simulink model "PEMFC"  (Simulink 8.3)
settings: Solver=ode45  StartTime=5.0  StopTime=20.0  RelTol=1e-3
settings Model: Creator=Cindy  LastModifiedBy=Cindy
settings DataIOCC: SaveState=on  SignalLoggingName=sigsOut
settings DebuggingCC: SaveWithParameterizedLinksMsg=none  SignalResolutionControl=TryResolveAllWithWarning  SolverPrmCheckMsg=none  MultiTaskDSMMsg=warning  MultiTaskCondExecSysMsg=none  StateNameClashWarn=none
settings HardwareCC: TargetUnknown=on
settings RTWCC: IncludeERTFirstTime=on

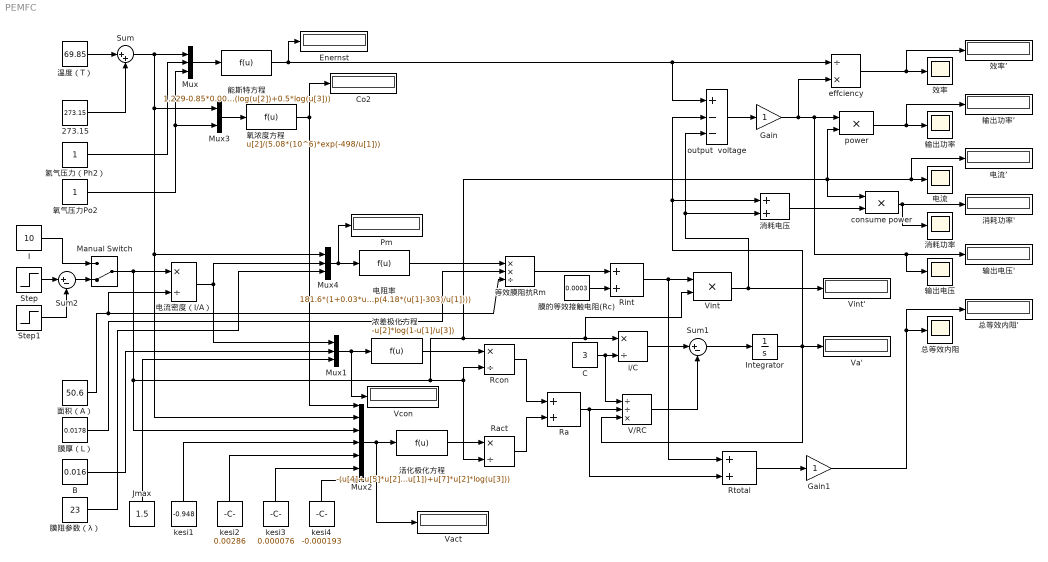
== system PEMFC ==
  273.15 : Constant  Value=273.15
  B : Constant  Value=0.016
  C : Constant  Value=3
  Co2 : Display
      settings: Format=short_e  Decimation=5
  Enernst : Display
      settings: Decimation=5
  Gain : Gain  SaturateOnIntegerOverflow=on  OutDataTypeStr=Inherit: Same as input  ParamDataTypeStr=Inherit: Same as input
  Gain1 : Gain  SaturateOnIntegerOverflow=on  OutDataTypeStr=Inherit: Same as input  ParamDataTypeStr=Inherit: Same as input
  I : Constant  Value=10
  Integrator : Integrator
  Jmax : Constant  Value=1.5
  Manual Switch : ManualSwitch  CurrentSetting=0
  Mux : Mux  Inputs=3
  Mux1 : Mux  Inputs=3
  Mux2 : Mux  Inputs=7
  Mux3 : Mux  Inputs=2
  Mux4 : Mux  Inputs=3
  Pm : Display
      settings: Decimation=5
  Ra : Sum  OutDataTypeStr=double
  Ract : Product  Inputs=*/  OutDataTypeStr=double
  Rcon : Product  Inputs=*/  OutDataTypeStr=double
  Rint : Sum  OutDataTypeStr=double
  Rtotal : Sum  OutDataTypeStr=double
  Step : Step  Time=10  Before=10  After=20  SampleTime=0
  Step1 : Step  Time=15  After=10  SampleTime=0
  Sum : Sum  Inputs=|++  SaturateOnIntegerOverflow=on
  Sum1 : Sum  Inputs=|+-  SaturateOnIntegerOverflow=on
  Sum2 : Sum  Inputs=|+-  SaturateOnIntegerOverflow=on
  V/RC : Product  Inputs=//*  OutDataTypeStr=double
  Va' : Display
      settings: Decimation=5
  Vact : Display
      settings: Decimation=5
  Vcon : Display
      settings: Decimation=5
  Vint : Product  SaturateOnIntegerOverflow=on  OutDataTypeStr=Inherit: Same as first input
  Vint' : Display
      settings: Decimation=5
  consume power : Product  SaturateOnIntegerOverflow=on  OutDataTypeStr=Inherit: Same as first input
  effciency : Product  Inputs=/*  OutDataTypeStr=double
  i/C : Product  Inputs=*/  OutDataTypeStr=double
  kesi1 : Constant  Value=-0.948
  kesi2 : Constant  Value=0.00286
  kesi3 : Constant  Value=0.000076
  kesi4 : Constant  Value=-0.000193
  output  voltage : Sum  Inputs=+--  OutDataTypeStr=double
  power : Product  SaturateOnIntegerOverflow=on  OutDataTypeStr=Inherit: Same as first input
  总等效内阻 : Scope
      settings: TimeRange=15  SaveName=ScopeData5
  总等效内阻' : Display
      settings: Decimation=5
  效率 : Scope
  效率’ : Display
      settings: Decimation=5
  氢气压力（Ph2） : Constant
  氧气压力Po2 : Constant
  氧浓度方程 : Fcn  Expr=u[2]/(5.08*(10^6)*exp(-498/u[1]))
  活化极化方程 : Fcn  Expr=-(u[4]+u[5]*u[2]+u[6]*u[2]*log(u[1])+u[7]*u[2]*log(u[3]))
  浓差极化方程 : Fcn  Expr=-u[2]*log(1-u[1]/u[3])
  消耗功率 : Scope
      settings: SaveName=ScopeData3
  消耗功率' : Display
      settings: Decimation=5
  消耗电压 : Sum  OutDataTypeStr=double
  温度（T） : Constant  Value=69.85
  电流 : Scope
  电流’ : Display
      settings: Decimation=5
  电流密度（I/A） : Product  Inputs=*/  OutDataTypeStr=double
  电阻率 : Fcn  Expr=181.6*(1+0.03*u[2]+0.062*((u[1]/303)^2)*(u[2]^2.5))/((u[3]-0.634-3*u[2])*(exp(4.18*(u[1]-303)/u[1])))
  等效膜阻抗Rm : Product  Inputs=**/  OutDataTypeStr=double
  能斯特方程 : Fcn  Expr=1.229-0.85*0.001*(u[1]-298.15)+4.3085*0.00001*u[1]*(log(u[2])+0.5*log(u[3]))
  膜厚（L） : Constant  Value=0.0178
  膜的等效接触电阻(Rc) : Constant  Value=0.0003
  膜阻参数（λ） : Constant  Value=23
  输出功率 : Scope
      settings: SaveName=ScopeData2
  输出功率’ : Display
      settings: Decimation=5
  输出电压 : Scope
      settings: SaveName=ScopeData4
  输出电压' : Display
      settings: Decimation=5
  面积（A） : Constant  Value=50.6
  wires:
  温度（T）/1 -> Sum/1
  273.15/1 -> Sum/2
  Sum/1 -> Mux/1, Mux3/1, Mux2/2, Mux4/1
  氧气压力Po2/1 -> Mux/3, Mux3/2
  氢气压力（Ph2）/1 -> Mux/2
  Mux/1 -> 能斯特方程/1
  能斯特方程/1 -> Enernst/1, effciency/1, output  voltage/1
  kesi1/1 -> Mux2/4
  kesi4/1 -> Mux2/7
  kesi3/1 -> Mux2/6
  kesi2/1 -> Mux2/5
  Mux3/1 -> 氧浓度方程/1
  氧浓度方程/1 -> Mux2/1, Co2/1
  Manual Switch/1 -> 电流密度（I/A）/1, Mux2/3, Ract/2, Rcon/2, i/C/1, Vint/2, power/2, consume power/1, 电流/1, 电流’/1
  面积（A）/1 -> 电流密度（I/A）/2, 等效膜阻抗Rm/3
  Mux2/1 -> 活化极化方程/1, Vact/1
  活化极化方程/1 -> Ract/1
  B/1 -> Mux1/2
  Jmax/1 -> Mux1/3
  电流密度（I/A）/1 -> Mux1/1, Mux4/2
  Mux1/1 -> 浓差极化方程/1, Vcon/1
  浓差极化方程/1 -> Rcon/1
  Rcon/1 -> Ra/1
  Ract/1 -> Ra/2
  膜阻参数（λ）/1 -> Mux4/3
  Mux4/1 -> 电阻率/1, Pm/1
  电阻率/1 -> 等效膜阻抗Rm/1
  膜厚（L）/1 -> 等效膜阻抗Rm/2
  等效膜阻抗Rm/1 -> Rint/1
  膜的等效接触电阻(Rc)/1 -> Rint/2
  C/1 -> i/C/2, V/RC/1
  Ra/1 -> V/RC/2, Rtotal/2
  i/C/1 -> Sum1/1
  V/RC/1 -> Sum1/2
  Sum1/1 -> Integrator/1
  Integrator/1 -> V/RC/3, Va'/1, output  voltage/2, 消耗电压/1
  Rint/1 -> Rtotal/1, Vint/1
  Vint/1 -> Vint'/1, output  voltage/3, 消耗电压/2
  Sum2/1 -> Manual Switch/2
  Step/1 -> Sum2/1
  Step1/1 -> Sum2/2
  I/1 -> Manual Switch/1
  消耗电压/1 -> consume power/2
  effciency/1 -> 效率/1, 效率’/1
  power/1 -> 输出功率/1, 输出功率’/1
  consume power/1 -> 消耗功率/1, 消耗功率'/1
  output  voltage/1 -> Gain/1
  Gain/1 -> effciency/2, power/1, 输出电压'/1, 输出电压/1
  Rtotal/1 -> Gain1/1
  Gain1/1 -> 总等效内阻'/1, 总等效内阻/1
